simulink subsystem "PvtSubSys_VSM_ELK"  (R2020b)
settings: Solver=VariableStepAuto  StartTime=0.0  StopTime=10.0  RelTol=1e-3
values from neighbouring files (symbols this model uses):
  P_VSM_ELK_Curvature_R_Table : value not decoded    [ELK.sldd]
  P_VSM_ELK_Curvature_R_Table_Calibration : value not decoded    [ELK.sldd]
  P_VSM_ELK_Lane_Width_Table : value not decoded    [ELK.sldd]
  P_VSM_ELK_Lane_Width_Table_Calibration : value not decoded    [ELK.sldd]
  P_VSM_ELK_Lateral_Speed_Table : value not decoded    [ELK.sldd]
  P_VSM_ELK_Lateral_Speed_Table_Calibration : value not decoded    [ELK.sldd]
  P_VSM_ELK_OnComing_Lateral = 2.8    [ELK.sldd]
  P_VSM_ELK_OnComing_TTC = 3.0    [ELK.sldd]
  P_VSM_ELK_OverTaking_Lateral = 2.0    [ELK.sldd]
  P_VSM_ELK_OverTaking_TTC = 5.0    [ELK.sldd]
  P_VSM_ELK_Sensitive_Table : value not decoded    [ELK.sldd]
  P_VSM_ELK_Sensitive_Table_Calibration : value not decoded    [ELK.sldd]
  P_VSM_ELK_State_Absesp_enable = 1.0    [ELK.sldd]
  P_VSM_ELK_State_Accpedalrate_enable = 1.0    [ELK.sldd]
  P_VSM_ELK_State_Breakpressure_enable = 1.0    [ELK.sldd]
  P_VSM_ELK_State_DriverInputTrqValue_enable = 1.0    [ELK.sldd]
  P_VSM_ELK_State_Eps_enable = 1.0    [ELK.sldd]
  P_VSM_ELK_State_ESSSts_enable = 1.0    [ELK.sldd]
  P_VSM_ELK_State_Failsafe_enable = 1.0    [ELK.sldd]
  P_VSM_ELK_State_GEAR_enable = 1.0    [ELK.sldd]
  P_VSM_ELK_State_Handson_enable = 1.0    [ELK.sldd]
  P_VSM_ELK_State_Headingangle_enable = 1.0    [ELK.sldd]
  P_VSM_ELK_State_Lane_enable = 1.0    [ELK.sldd]
  P_VSM_ELK_State_LaneChange_enable = 1.0    [ELK.sldd]
  P_VSM_ELK_State_Lanecurve_enable = 1.0    [ELK.sldd]
  P_VSM_ELK_State_LateralAcce_enable = 1.0    [ELK.sldd]
  P_VSM_ELK_State_LongitudeAcc_enable = 1.0    [ELK.sldd]
  P_VSM_ELK_State_Overide_enable = 1.0    [ELK.sldd]
  P_VSM_ELK_State_Param_AngleOffset = 0.05    [ELK.sldd]
  P_VSM_ELK_State_Param_LaneTime : value not decoded    [ELK.sldd]
  P_VSM_ELK_State_Param_Oncoming = 0.55    [ELK.sldd]
  P_VSM_ELK_State_Param_OnTime : value not decoded    [ELK.sldd]
  P_VSM_ELK_State_Param_OutOffset = 0.15    [ELK.sldd]
  P_VSM_ELK_State_Param_Over = 0.55    [ELK.sldd]
  P_VSM_ELK_State_Param_OvTime : value not decoded    [ELK.sldd]
  P_VSM_ELK_State_Param_Speed : value not decoded    [ELK.sldd]
  P_VSM_ELK_State_SteerWheelAngle_enable = 1.0    [ELK.sldd]
  P_VSM_ELK_State_SteerWheelSpd_enable = 1.0    [ELK.sldd]
  P_VSM_ELK_State_TurnLight_enable = 1.0    [ELK.sldd]
  P_VSM_ELK_State_Vehspeed_enable = 1.0    [ELK.sldd]
  P_VSM_ELK_State_Yawsup_enable = 1.0    [ELK.sldd]
undefined symbols (not defined in the file or in its folder): ELKSTATE, P_Global_DxvRearBumper_m, P_Global_IEnvironment_RefPX_Front_Bumper, P_Global_IFV2Fwheel_Dx, P_Global_Vehicle_Length_m, P_Global_VehicleWidthMin_m, P_VSM_LSMC_SampleTime
libraries: simulink x167
(part 3 of 5)

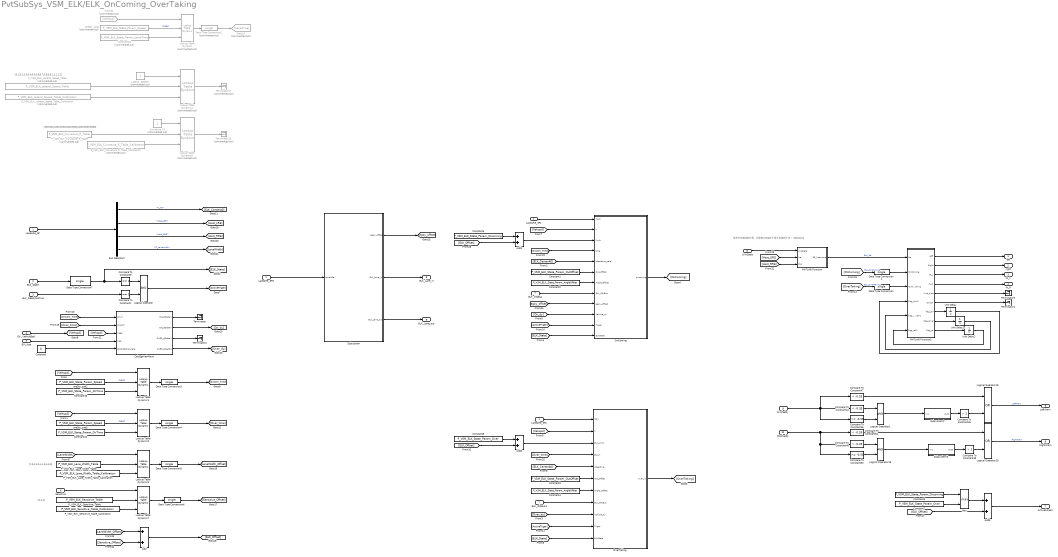
== system PvtSubSys_VSM_ELK/ELK_OnComing_OverTaking ==
  note: 目前对车道线起作用，但是ELKState不显示车道线干涉；
      | 20201011
  note: [0,1,2]
  note: [0.1,0.2,0.3,0.4,0.5,0.6,0.7,0.8,0.9,1,1.1,1.2]
  note: [2.5,3,3.5,4,4.5,5,5.5]
  note: [150,500,1000,1500,2000,3000,4000,5000,5500]
  LaneARe_SP : Inport
  ELK_State : Inport  Port=2
  ELK_Ready2Active : Inport  Port=3
  EVI_VehicleSpd : Inport  Port=4
  EVI_Kap : Inport  Port=5
  Sensitive : Inport  Port=6
  ELK_ObjBus : Inport  Port=7
  LKAState : Inport  Port=8
  FLWhelDy : Inport  Port=9
  FRWhelDy : Inport  Port=10
  Add{,1..3} (4 alike) : Sum
  Bus Selector2 : BusSelector  OutputSignals=T_A0,Host_LRE,Host_RRE,C_Lanewidth
  CalcEgoVehMove : MATLAB Function  TreatAsAtomicUnit=on
  Compare To Constant1 : simulink/Logic and Bit Operations/Compare To Constant  relop===  const=1  OutDataTypeStr=boolean
  Compare To Constant44 : simulink/Logic and Bit Operations/Compare To Constant  relop=<  const=-0.35  OutDataTypeStr=boolean
  Compare To Constant45 : simulink/Logic and Bit Operations/Compare To Constant  relop=>  const=2  OutDataTypeStr=boolean
  Compare To Constant46 : simulink/Logic and Bit Operations/Compare To Constant  relop=>=  const=-0.55  OutDataTypeStr=boolean
  Compare To Constant47 : simulink/Logic and Bit Operations/Compare To Constant  relop=<  const=-0.55  OutDataTypeStr=boolean
  Compare To Constant48 : simulink/Logic and Bit Operations/Compare To Constant  relop=<  const=-0.35  OutDataTypeStr=boolean
  Compare To Constant49 : simulink/Logic and Bit Operations/Compare To Constant  relop=>  const=2  OutDataTypeStr=boolean
  Compare To Constant50 : simulink/Logic and Bit Operations/Compare To Constant  relop=>=  const=-0.55  OutDataTypeStr=boolean
  Compare To Constant51 : simulink/Logic and Bit Operations/Compare To Constant  relop=<  const=-0.55  OutDataTypeStr=boolean
  Compare To Constant9 : simulink/Logic and Bit Operations/Compare To Constant  relop===  const=2  OutDataTypeStr=boolean
  Constant : Constant  Value=0  OutDataTypeStr=single
  Constant1 : Constant  Value=P_VSM_ELK_State_Param_OutOffset
  Constant10 : Constant  Value=P_VSM_ELK_State_Param_OvTime
  Constant15 : Constant  Commented=on  Value=P_VSM_ELK_State_Param_LaneTime
  Constant16 : Constant  Value=P_VSM_ELK_State_Param_OnTime
  Constant2 : Constant  Value=P_VSM_ELK_State_Param_AngleOffset
  Constant3 : Constant  Value=P_VSM_ELK_State_Param_OutOffset
  Constant4 : Constant  Value=P_VSM_ELK_State_Param_AngleOffset
  Constant5 : Constant  Value=P_VSM_ELK_State_Param_Oncoming
  Constant6 : Constant  Value=P_VSM_ELK_State_Param_Oncoming
  Constant7 : Constant  Value=P_VSM_ELK_State_Param_Over
  Constant8 : Constant  Value=P_VSM_ELK_State_Param_Over
  Curvature_R1 : Constant  Commented=on
  Data Type Conversion{,1,3..7} (7 alike) : DataTypeConversion  OutDataTypeStr=single
  Data Type Conversion2 : DataTypeConversion  Commented=on  OutDataTypeStr=single
  ELK_ObjBus1 : InportShadow  Port=7
  From21 : From  Commented=on  GotoTag=VehSpd
  Goto14 : Goto  Commented=on  GotoTag=LaneTime
  LaneARe_SP1 : InportShadow
  LaneARe_SP2 : InportShadow
  LaneARe_SP3 : InportShadow
  Lateral_Speed1 : Constant  Commented=on
  Logical Operator : Logic  AllPortsSameDT=off  OutDataTypeStr=boolean
  Logical Operator1 : Logic  AllPortsSameDT=off  OutDataTypeStr=boolean
  Logical Operator18 : Logic  Operator=OR  AllPortsSameDT=off  OutDataTypeStr=boolean
  Logical Operator19 : Logic  AllPortsSameDT=off  OutDataTypeStr=boolean
  Logical Operator20 : Logic  Operator=OR  AllPortsSameDT=off  OutDataTypeStr=boolean
  Lookup Table Dynamic : simulink/Lookup Tables/Lookup Table Dynamic  Commented=on  LookUpMeth=Interpolation-Use End Values  OutDataType=fixdt('double')  OutScaling=[]  OutputDataTypeScalingMode=Specify via dialog  OutDataTypeStr=double  DoSatur=off
  Lookup Table Dynamic{1..2,5,7} (4 alike) : simulink/Lookup Tables/Lookup Table Dynamic  LookUpMeth=Interpolation-Use End Values  OutDataType=fixdt('double')  OutScaling=[]  OutputDataTypeScalingMode=Specify via dialog  OutDataTypeStr=double  DoSatur=off
  Lookup Table Dynamic4 : simulink/Lookup Tables/Lookup Table Dynamic  Commented=on  LookUpMeth=Interpolation-Use End Values  OutDataType=fixdt('double')  OutScaling=[]  OutputDataTypeScalingMode=Specify via dialog  OutDataTypeStr=double  DoSatur=off
  Lookup Table Dynamic6 : simulink/Lookup Tables/Lookup Table Dynamic  Commented=on  LookUpMeth=Interpolation-Use End Values  OutDataType=fixdt('double')  OutScaling=[]  OutputDataTypeScalingMode=Specify via dialog  OutDataTypeStr=double  DoSatur=off
  MATLAB Function : MATLAB Function  TreatAsAtomicUnit=on
  MATLAB Function2 : MATLAB Function  TreatAsAtomicUnit=on
  Max : MinMax  Function=max  Inputs=2
  OnComing : Subsystem
  OverTaking : Subsystem
  P_VSM_ELK_Curvature_R_Table : Constant  Commented=on  Value=P_VSM_ELK_Curvature_R_Table
  P_VSM_ELK_Curvature_R_Table_Calibration : Constant  Commented=on  Value=P_VSM_ELK_Curvature_R_Table_Calibration
  P_VSM_ELK_Lane_Width_Table : Constant  Value=P_VSM_ELK_Lane_Width_Table
  P_VSM_ELK_Lane_Width_Table_Calibration : Constant  Value=P_VSM_ELK_Lane_Width_Table_Calibration
  P_VSM_ELK_Lateral_Speed_Table : Constant  Commented=on  Value=P_VSM_ELK_Lateral_Speed_Table
  P_VSM_ELK_Lateral_Speed_Table_Calibration : Constant  Commented=on  Value=P_VSM_ELK_Lateral_Speed_Table_Calibration
  P_VSM_ELK_Sensitive_Table : Constant  Value=P_VSM_ELK_Sensitive_Table
  P_VSM_ELK_Sensitive_Table_Calibration : Constant  Value=P_VSM_ELK_Sensitive_Table_Calibration
  Subsystem : Subsystem
  Subsystem2 : Subsystem  mask{Ts=P_VSM_LSMC_SampleTime, Max=10}
      mask prompts: Ts "Sample Time:"; Max "Max Limit:"
      mask Display:
      | Ts=get_param(gcb,'Ts');
      | Max=get_param(gcb,'Max');
      | disp(['Ts:' Ts '\n' 'Max:' Max ]);
  Subsystem3 : Subsystem  mask{Ts=P_VSM_LSMC_SampleTime, Max=10}
      mask prompts: Ts "Sample Time:"; Max "Max Limit:"
      mask Display:
      | Ts=get_param(gcb,'Ts');
      | Max=get_param(gcb,'Max');
      | disp(['Ts:' Ts '\n' 'Max:' Max ]);
  Terminator{,1..3} (4 alike) : Terminator
  Terminator11 : Terminator  Commented=on
  Terminator13 : Terminator  Commented=on
  Unit Delay : UnitDelay  SampleTime=-1  HasFrameUpgradeWarning=on
  Unit Delay1 : UnitDelay  InitialCondition=single(0)  SampleTime=-1  HasFrameUpgradeWarning=on
  Unit Delay2 : UnitDelay  InitialCondition=single(0)  SampleTime=-1  HasFrameUpgradeWarning=on
  preDis_spd1 : Constant  Commented=on  Value=P_VSM_ELK_State_Param_Speed
  preDis_spd2 : Constant  Value=P_VSM_ELK_State_Param_Speed
  preDis_spd3 : Constant  Value=P_VSM_ELK_State_Param_Speed
  "left " : Outport
  "right " : Outport  Port=2
  IN_L : Outport  Port=3
  IN_R : Outport  Port=4
  LeftWarn : Outport  Port=5
  RightWarn : Outport  Port=6
  ActiveZoneIn : Outport  Port=7
  ELK_Lane_in : Outport  Port=8
  ELK_Lane_out : Outport  Port=9
  wires:
  Data Type Conversion7/1 -> [ELK_State], Compare To Constant9/1
  LaneARe_SP2/1 -> OverTaking/1(ican)
  LaneARe_SP1/1 -> OnComing/1(ICAN)
  [On_dy] -> OnComing/10(Vehicle_dy)
  [Over_dy] -> OverTaking/9(Vehicle_dy)
  OverTaking/1("over_in ") -> [OverTaking]
  OnComing/1(oncoming) -> [OnComing]
  ELK_ObjBus1/1 -> OverTaking/8(ELK_ObjBus)
  ELK_ObjBus/1 -> OnComing/8(ELK_ObjBus)
  LKAState/1 -> MATLAB Function/1(LKAState)
  [OnComing] -> Data Type Conversion1/1  "ELK_OnComing"
  [OverTaking] -> Data Type Conversion/1  "ELK_OverTaking"
  MATLAB Function2/6(Switch) -> Terminator1/1
  MATLAB Function2/5(Line_type) -> Terminator3/1
  [egoy_offset] -> OnComing/9(egoy_offset)
  MATLAB Function2/1(Left) -> "left "/1
  MATLAB Function2/2(Right) -> "right "/1
  MATLAB Function2/3(IN_L) -> IN_L/1
  MATLAB Function2/4(IN_R) -> IN_R/1
  Constant1/1 -> OnComing/6(Out_Offset)
  Constant2/1 -> OnComing/7(Angle_Offset)
  [ELK_CenterA0] -> OverTaking/5(Ldeactive)
  Constant3/1 -> OverTaking/6(Out_Offset)
  Constant4/1 -> OverTaking/7(Angle_Offset)
  MATLAB Function2/7(flag_On) -> Unit Delay/1
  MATLAB Function2/8(flag_Over) -> Unit Delay1/1
  MATLAB Function2/9(flag_re) -> Unit Delay2/1
  Unit Delay/1 -> MATLAB Function2/4(flag_Onk1)
  Unit Delay1/1 -> MATLAB Function2/5(flag_Overk1)
  Unit Delay2/1 -> MATLAB Function2/6(flag_rek1)
  MATLAB Function/1(RE_Intervene) -> MATLAB Function2/1(Re)  "ELK_Re"
  [Host_LRE] -> MATLAB Function/2(Lre)
  [Host_RRE] -> MATLAB Function/3(Rre)
  LaneARe_SP/1 -> Bus Selector2/1
  [ELK_CenterA0] -> OnComing/5(Ldeactive_para)
  [ActiveTriger] -> OnComing/11(Triger)
  [ActiveTriger] -> OverTaking/10(Triger)
  Compare To Constant9/1 -> Logical Operator/1
  Compare To Constant1/1 -> Logical Operator/2
  ELK_State/1 -> Data Type Conversion7/1
  ELK_Ready2Active/1 -> Compare To Constant1/1
  Logical Operator/1 -> [ActiveTriger]
  [ELK_State] -> OnComing/12(ELKState)
  [ELK_State] -> OverTaking/11(ELKState)
  Compare To Constant46/1 -> Logical Operator1/2
  Compare To Constant50/1 -> Logical Operator19/2
  Compare To Constant47/1 -> Logical Operator18/1
  Compare To Constant48/1 -> Logical Operator19/1
  Compare To Constant51/1 -> Logical Operator20/1
  FRWhelDy/1 -> Compare To Constant48/1, Compare To Constant50/1, Compare To Constant51/1
  Logical Operator19/1 -> Subsystem3/1(In1)
  Compare To Constant49/1 -> Logical Operator20/2
  Subsystem2/1(Out1) -> Compare To Constant45/1
  Compare To Constant44/1 -> Logical Operator1/1
  Compare To Constant45/1 -> Logical Operator18/2
  FLWhelDy/1 -> Compare To Constant46/1, Compare To Constant47/1, Compare To Constant44/1
  Logical Operator1/1 -> Subsystem2/1(In1)
  Subsystem3/1(Out1) -> Compare To Constant49/1
  Logical Operator18/1 -> LeftWarn/1  "LeftWarn"
  Logical Operator20/1 -> RightWarn/1  "RightWarn"
  Data Type Conversion/1 -> MATLAB Function2/3(OverTaking)
  Data Type Conversion1/1 -> MATLAB Function2/2(OnComing)
  [Vehspd] -> OnComing/2(V)
  [Vehspd] -> OverTaking/2(V)
  EVI_Kap/1 -> CalcEgoVehMove/4(Kap)
  Constant/1 -> CalcEgoVehMove/5(alpSideSlipAngle)
  [Vehspd] -> CalcEgoVehMove/3(Vego)
  [Oncom_Time] -> CalcEgoVehMove/1(On_T)
  [Over_time] -> CalcEgoVehMove/2(Over_T)
  [Oncom_Time] -> OnComing/4(time)
  [Over_time] -> OverTaking/4(ELK_T)
  CalcEgoVehMove/2(ON_dDeltaY) -> [On_dy]
  CalcEgoVehMove/4(OVER_dDeltaY) -> [Over_dy]
  CalcEgoVehMove/1(ON_dDeltaX) -> Terminator/1
  CalcEgoVehMove/3(OVER_dDeltaX) -> Terminator2/1
  EVI_VehicleSpd/1 -> [Vehspd]
  preDis_spd3/1 -> Lookup Table Dynamic2/2  "speed"
  Data Type Conversion3/1 -> [Oncom_Time]
  [Vehspd] -> Lookup Table Dynamic2/1
  preDis_spd1/1 -> Lookup Table Dynamic/2  "speed"
  Lookup Table Dynamic/1 -> Data Type Conversion2/1
  Constant15/1 -> Lookup Table Dynamic/3
  Lookup Table Dynamic1/1 -> Data Type Conversion3/1
  From21/1 -> Lookup Table Dynamic/1
  Constant16/1 -> Lookup Table Dynamic1/3
  Lookup Table Dynamic2/1 -> Data Type Conversion4/1
  Data Type Conversion4/1 -> [Over_time]
  Constant10/1 -> Lookup Table Dynamic2/3
  preDis_spd2/1 -> Lookup Table Dynamic1/2  "speed"
  Data Type Conversion2/1 -> Goto14/1
  [Vehspd] -> Lookup Table Dynamic1/1
  Bus Selector2/1 -> [ELK_CenterA0]  "<T_A0>"
  Constant6/1 -> Add1/1
  [ELK_Offset] -> Add2/2
  [ELK_Offset] -> Add1/2
  Add/1 -> [ELK_Offset]
  Sensitive/1 -> Lookup Table Dynamic7/1
  Data Type Conversion5/1 -> [LaneWidth_Offset]
  P_VSM_ELK_Sensitive_Table/1 -> Lookup Table Dynamic7/2
  Data Type Conversion6/1 -> [Sensitive_Offset]
  [LaneWidth] -> Lookup Table Dynamic5/1
  Lookup Table Dynamic5/1 -> Data Type Conversion5/1
  Lookup Table Dynamic6/1 -> Terminator13/1
  P_VSM_ELK_Lane_Width_Table/1 -> Lookup Table Dynamic5/2
  P_VSM_ELK_Lateral_Speed_Table_Calibration/1 -> Lookup Table Dynamic4/3
  [LaneWidth_Offset] -> Add/1
  P_VSM_ELK_Sensitive_Table_Calibration/1 -> Lookup Table Dynamic7/3
  [Sensitive_Offset] -> Add/2
  P_VSM_ELK_Curvature_R_Table/1 -> Lookup Table Dynamic6/2
  P_VSM_ELK_Curvature_R_Table_Calibration/1 -> Lookup Table Dynamic6/3
  Lookup Table Dynamic4/1 -> Terminator11/1
  Curvature_R1/1 -> Lookup Table Dynamic6/1
  Lateral_Speed1/1 -> Lookup Table Dynamic4/1
  P_VSM_ELK_Lane_Width_Table_Calibration/1 -> Lookup Table Dynamic5/3
  Lookup Table Dynamic7/1 -> Data Type Conversion6/1
  P_VSM_ELK_Lateral_Speed_Table/1 -> Lookup Table Dynamic4/2
  Add1/1 -> OnComing/3(limit)
  Constant8/1 -> Add2/1
  Add2/1 -> OverTaking/3(ELK_Limit)
  Bus Selector2/2 -> [Host_LRE]  "<Host_LRE>"
  Bus Selector2/3 -> [Host_RRE]  "<Host_RRE>"
  Bus Selector2/4 -> [LaneWidth]  "<C_Lanewidth>"
  Constant5/1 -> Max/1
  Constant7/1 -> Max/2
  Max/1 -> Add3/1
  [ELK_Offset] -> Add3/2
  Add3/1 -> ActiveZoneIn/1
  Subsystem/1(egoy_offset) -> [egoy_offset]
  Subsystem/2(ELK_Lane_in) -> ELK_Lane_in/1
  Subsystem/3(ELK_Lane_out) -> ELK_Lane_out/1
  LaneARe_SP3/1 -> Subsystem/1(LaneARe)

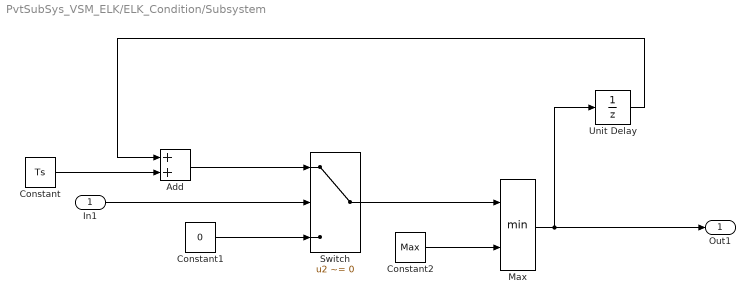
== system PvtSubSys_VSM_ELK/ELK_Condition/Subsystem ==
  In1 : Inport
  Add : Sum
  Constant : Constant  Value=Ts
  Constant1 : Constant  Value=0
  Constant2 : Constant  Value=Max
  Max : MinMax  Inputs=2
  Switch : Switch  Criteria=u2 ~= 0
  Unit Delay : UnitDelay  SampleTime=-1  HasFrameUpgradeWarning=on
  Out1 : Outport
  wires:
  Switch/1 -> Max/1
  Constant2/1 -> Max/2
  Max/1 -> Out1/1, Unit Delay/1
  Add/1 -> Switch/1
  Constant1/1 -> Switch/3
  Constant/1 -> Add/2
  In1/1 -> Switch/2
  Unit Delay/1 -> Add/1

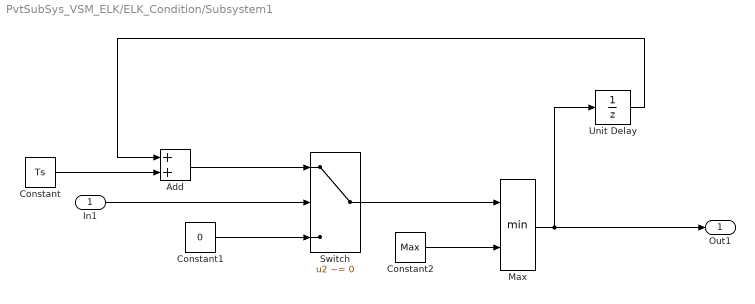
== system PvtSubSys_VSM_ELK/ELK_Condition/Subsystem1 ==
  In1 : Inport
  Add : Sum
  Constant : Constant  Value=Ts
  Constant1 : Constant  Value=0  OutDataTypeStr=single
  Constant2 : Constant  Value=Max  OutDataTypeStr=single
  Max : MinMax  Inputs=2
  Switch : Switch  Criteria=u2 ~= 0
  Unit Delay : UnitDelay  SampleTime=-1  HasFrameUpgradeWarning=on
  Out1 : Outport
  wires:
  Unit Delay/1 -> Add/1
  In1/1 -> Switch/2
  Constant/1 -> Add/2
  Constant1/1 -> Switch/3
  Add/1 -> Switch/1
  Max/1 -> Unit Delay/1, Out1/1
  Constant2/1 -> Max/2
  Switch/1 -> Max/1

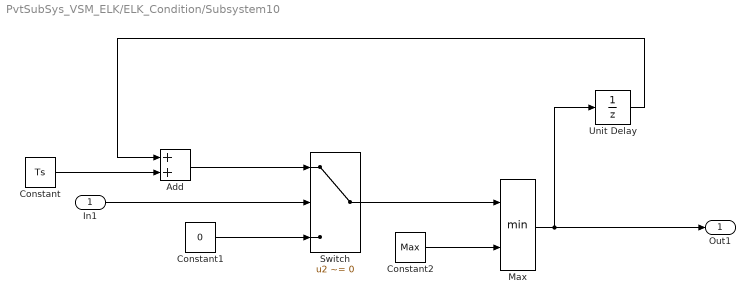
== system PvtSubSys_VSM_ELK/ELK_Condition/Subsystem10 ==
  In1 : Inport
  Add : Sum
  Constant : Constant  Value=Ts
  Constant1 : Constant  Value=0
  Constant2 : Constant  Value=Max
  Max : MinMax  Inputs=2
  Switch : Switch  Criteria=u2 ~= 0
  Unit Delay : UnitDelay  SampleTime=-1  HasFrameUpgradeWarning=on
  Out1 : Outport
  wires:
  Unit Delay/1 -> Add/1
  In1/1 -> Switch/2
  Constant/1 -> Add/2
  Constant1/1 -> Switch/3
  Add/1 -> Switch/1
  Max/1 -> Unit Delay/1, Out1/1
  Constant2/1 -> Max/2
  Switch/1 -> Max/1

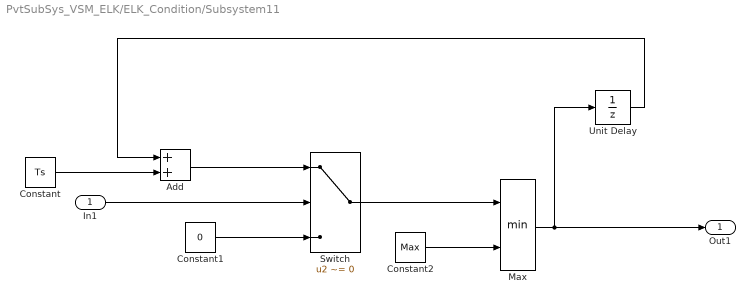
== system PvtSubSys_VSM_ELK/ELK_Condition/Subsystem11 ==
  In1 : Inport
  Add : Sum
  Constant : Constant  Value=Ts
  Constant1 : Constant  Value=0
  Constant2 : Constant  Value=Max
  Max : MinMax  Inputs=2
  Switch : Switch  Criteria=u2 ~= 0
  Unit Delay : UnitDelay  SampleTime=-1  HasFrameUpgradeWarning=on
  Out1 : Outport
  wires:
  Switch/1 -> Max/1
  Constant2/1 -> Max/2
  Max/1 -> Out1/1, Unit Delay/1
  Add/1 -> Switch/1
  Constant1/1 -> Switch/3
  Constant/1 -> Add/2
  In1/1 -> Switch/2
  Unit Delay/1 -> Add/1

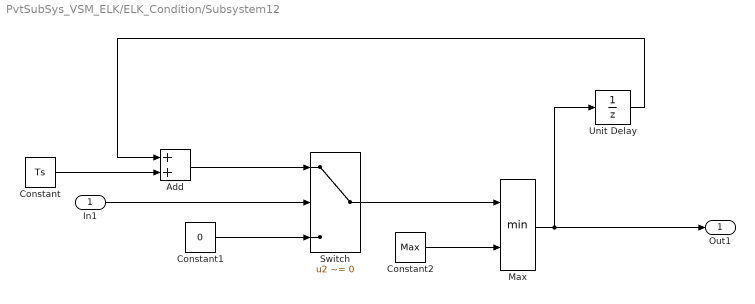
== system PvtSubSys_VSM_ELK/ELK_Condition/Subsystem12 ==
  In1 : Inport
  Add : Sum
  Constant : Constant  Value=Ts
  Constant1 : Constant  Value=0
  Constant2 : Constant  Value=Max
  Max : MinMax  Inputs=2
  Switch : Switch  Criteria=u2 ~= 0
  Unit Delay : UnitDelay  SampleTime=-1  HasFrameUpgradeWarning=on
  Out1 : Outport
  wires:
  Switch/1 -> Max/1
  Constant2/1 -> Max/2
  Max/1 -> Out1/1, Unit Delay/1
  Add/1 -> Switch/1
  Constant1/1 -> Switch/3
  Constant/1 -> Add/2
  In1/1 -> Switch/2
  Unit Delay/1 -> Add/1

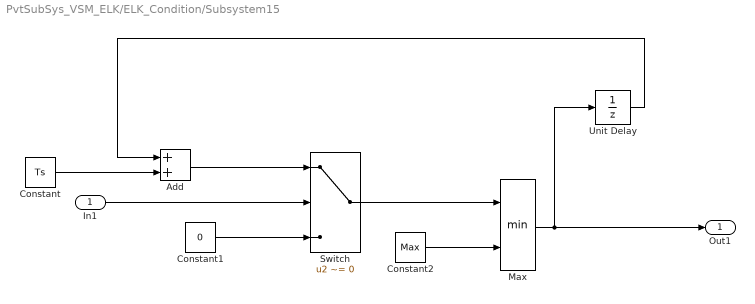
== system PvtSubSys_VSM_ELK/ELK_Condition/Subsystem15 ==
  In1 : Inport
  Add : Sum
  Constant : Constant  Value=Ts
  Constant1 : Constant  Value=0
  Constant2 : Constant  Value=Max
  Max : MinMax  Inputs=2
  Switch : Switch  Criteria=u2 ~= 0
  Unit Delay : UnitDelay  SampleTime=-1  HasFrameUpgradeWarning=on
  Out1 : Outport
  wires:
  Switch/1 -> Max/1
  Constant2/1 -> Max/2
  Max/1 -> Out1/1, Unit Delay/1
  Add/1 -> Switch/1
  Constant1/1 -> Switch/3
  Constant/1 -> Add/2
  In1/1 -> Switch/2
  Unit Delay/1 -> Add/1

== system PvtSubSys_VSM_ELK/ELK_Condition/Subsystem17 ==
  In1 : Inport
  Add : Sum
  Constant : Constant  Value=Ts
  Constant1 : Constant  Value=0
  Constant2 : Constant  Value=Max
  Max : MinMax  Inputs=2
  Switch : Switch  Criteria=u2 ~= 0
  Unit Delay : UnitDelay  SampleTime=-1  HasFrameUpgradeWarning=on
  Out1 : Outport
  wires:
  Unit Delay/1 -> Add/1
  In1/1 -> Switch/2
  Constant/1 -> Add/2
  Constant1/1 -> Switch/3
  Add/1 -> Switch/1
  Max/1 -> Unit Delay/1, Out1/1
  Constant2/1 -> Max/2
  Switch/1 -> Max/1

== system PvtSubSys_VSM_ELK/ELK_Condition/Subsystem2 ==
  In1 : Inport
  Add : Sum
  Constant : Constant  Value=Ts
  Constant1 : Constant  Value=0
  Constant2 : Constant  Value=Max
  Max : MinMax  Inputs=2
  Switch : Switch  Criteria=u2 ~= 0
  Unit Delay : UnitDelay  SampleTime=-1  HasFrameUpgradeWarning=on
  Out1 : Outport
  wires:
  Switch/1 -> Max/1
  Constant2/1 -> Max/2
  Max/1 -> Out1/1, Unit Delay/1
  Add/1 -> Switch/1
  Constant1/1 -> Switch/3
  Constant/1 -> Add/2
  In1/1 -> Switch/2
  Unit Delay/1 -> Add/1

== system PvtSubSys_VSM_ELK/ELK_Condition/Subsystem4 ==
  In1 : Inport
  Add : Sum
  Constant : Constant  Value=Ts
  Constant1 : Constant  Value=0
  Constant2 : Constant  Value=Max
  Max : MinMax  Inputs=2
  Switch : Switch  Criteria=u2 ~= 0
  Unit Delay : UnitDelay  SampleTime=-1  HasFrameUpgradeWarning=on
  Out1 : Outport
  wires:
  Unit Delay/1 -> Add/1
  In1/1 -> Switch/2
  Constant/1 -> Add/2
  Constant1/1 -> Switch/3
  Add/1 -> Switch/1
  Max/1 -> Unit Delay/1, Out1/1
  Constant2/1 -> Max/2
  Switch/1 -> Max/1

== system PvtSubSys_VSM_ELK/ELK_Condition/Subsystem5 ==
  In1 : Inport
  Add : Sum
  Constant : Constant  Value=Ts
  Constant1 : Constant  Value=0
  Constant2 : Constant  Value=Max
  Max : MinMax  Inputs=2
  Switch : Switch  Criteria=u2 ~= 0
  Unit Delay : UnitDelay  SampleTime=-1  HasFrameUpgradeWarning=on
  Out1 : Outport
  wires:
  Switch/1 -> Max/1
  Constant2/1 -> Max/2
  Max/1 -> Out1/1, Unit Delay/1
  Add/1 -> Switch/1
  Constant1/1 -> Switch/3
  Constant/1 -> Add/2
  In1/1 -> Switch/2
  Unit Delay/1 -> Add/1

== system PvtSubSys_VSM_ELK/ELK_Condition/Subsystem6 ==
  In1 : Inport
  Add : Sum
  Constant : Constant  Value=Ts
  Constant1 : Constant  Value=0
  Constant2 : Constant  Value=Max
  Max : MinMax  Inputs=2
  Switch : Switch  Criteria=u2 ~= 0
  Unit Delay : UnitDelay  SampleTime=-1  HasFrameUpgradeWarning=on
  Out1 : Outport
  wires:
  Switch/1 -> Max/1
  Constant2/1 -> Max/2
  Max/1 -> Out1/1, Unit Delay/1
  Add/1 -> Switch/1
  Constant1/1 -> Switch/3
  Constant/1 -> Add/2
  In1/1 -> Switch/2
  Unit Delay/1 -> Add/1

== system PvtSubSys_VSM_ELK/ELK_Condition/Subsystem7 ==
  In1 : Inport
  Add : Sum
  Constant : Constant  Value=Ts
  Constant1 : Constant  Value=0
  Constant2 : Constant  Value=Max
  Max : MinMax  Inputs=2
  Switch : Switch  Criteria=u2 ~= 0
  Unit Delay : UnitDelay  SampleTime=-1  HasFrameUpgradeWarning=on
  Out1 : Outport
  wires:
  Unit Delay/1 -> Add/1
  In1/1 -> Switch/2
  Constant/1 -> Add/2
  Constant1/1 -> Switch/3
  Add/1 -> Switch/1
  Max/1 -> Unit Delay/1, Out1/1
  Constant2/1 -> Max/2
  Switch/1 -> Max/1

== system PvtSubSys_VSM_ELK/ELK_Condition/Subsystem8 ==
  In1 : Inport
  Add : Sum
  Constant : Constant  Value=Ts
  Constant1 : Constant  Value=0
  Constant2 : Constant  Value=Max
  Max : MinMax  Inputs=2
  Switch : Switch  Criteria=u2 ~= 0
  Unit Delay : UnitDelay  SampleTime=-1  HasFrameUpgradeWarning=on
  Out1 : Outport
  wires:
  Unit Delay/1 -> Add/1
  In1/1 -> Switch/2
  Constant/1 -> Add/2
  Constant1/1 -> Switch/3
  Add/1 -> Switch/1
  Max/1 -> Unit Delay/1, Out1/1
  Constant2/1 -> Max/2
  Switch/1 -> Max/1

== system PvtSubSys_VSM_ELK/ELK_Condition/Subsystem9 ==
  In1 : Inport
  Add : Sum
  Constant : Constant  Value=Ts
  Constant1 : Constant  Value=0
  Constant2 : Constant  Value=Max
  Max : MinMax  Inputs=2
  Switch : Switch  Criteria=u2 ~= 0
  Unit Delay : UnitDelay  SampleTime=-1  HasFrameUpgradeWarning=on
  Out1 : Outport
  wires:
  Switch/1 -> Max/1
  Constant2/1 -> Max/2
  Max/1 -> Out1/1, Unit Delay/1
  Add/1 -> Switch/1
  Constant1/1 -> Switch/3
  Constant/1 -> Add/2
  In1/1 -> Switch/2
  Unit Delay/1 -> Add/1

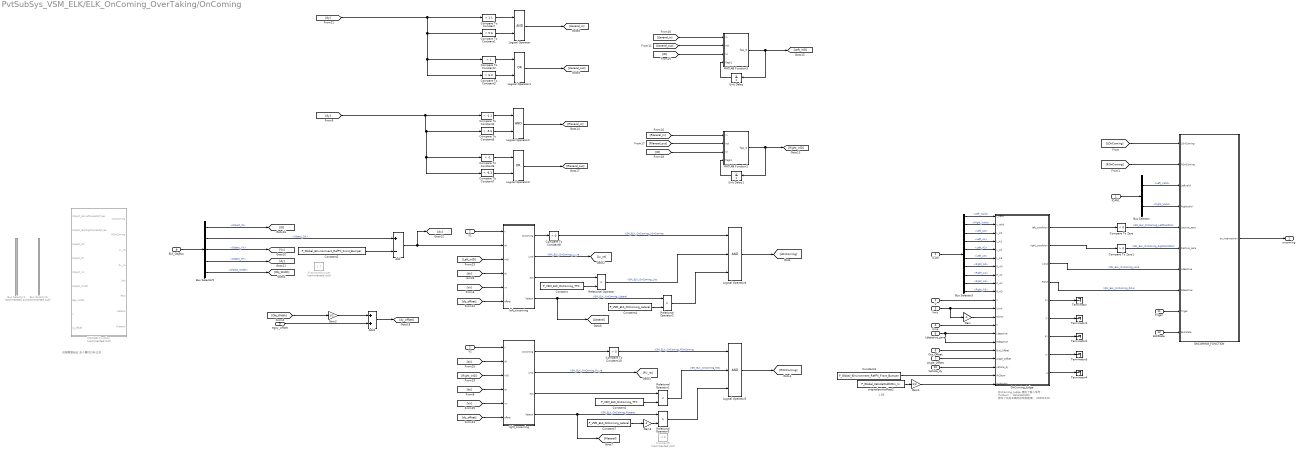
== system PvtSubSys_VSM_ELK/ELK_OnComing_OverTaking/OnComing ==
  note: OnComing_Judge
      | 增加了输入信号：
      | ifv2bum；
      | VehicleWidth;
      | 修改了自车车辆动态预测距离；
      | 20201010
  note: 后期需要验证 各个属性方向/正负
  note: 1.86
  ICAN : Inport
  V : Inport  Port=2
  limit : Inport  Port=3
  time : Inport  Port=4
  Ldeactive_para : Inport  Port=5
  Out_Offset : Inport  Port=6
  Angle_Offset : Inport  Port=7
  ELK_ObjBus : Inport  Port=8
  egoy_offset : Inport  Port=9
  Vehicle_dy : Inport  Port=10
  Triger : Inport  Port=11
  ELKState : Inport  Port=12
  Add : Sum  Inputs=+-
  Add1 : Sum
  Bus Selector : BusSelector  OutputSignals=Left_Valid,Right_Valid
  Bus Selector1 : BusSelector  Commented=on  OutputSignals=ELK_Object_ID,ELK_Object_DX,ELK_Object_VX,ELK_Object_DY,ELK_Object_Width
  Bus Selector3 : BusSelector  OutputSignals=Left_Valid,Right_Valid,Left_A0,Left_A1,Left_A2,Left_A3,Right_A0,Right_A1,Right_A2,Right_A3
  Bus Selector5 : BusSelector  OutputSignals=Object_ID,Object_DX,Object_VX,Object_DY,Object_Width
  Bus Selector6 : BusSelector  Commented=on  OutputSignals=IFC_ID,Long_Pos,Long_Vel,Lat_Pos,VIS_OBS_WIDTH
  Compare To Constant : simulink/Logic and Bit Operations/Compare To Constant  relop=>  const=1.1  OutDataTypeStr=boolean
  Compare To Constant1 : simulink/Logic and Bit Operations/Compare To Constant  relop=<  const=5.6  OutDataTypeStr=boolean
  Compare To Constant10 : simulink/Logic and Bit Operations/Compare To Constant  relop=>  const=0  OutDataTypeStr=boolean
  Compare To Constant2 : simulink/Logic and Bit Operations/Compare To Constant  relop=<  const=1  OutDataTypeStr=boolean
  Compare To Constant3 : simulink/Logic and Bit Operations/Compare To Constant  relop=>  const=6.3  OutDataTypeStr=boolean
  Compare To Constant4 : simulink/Logic and Bit Operations/Compare To Constant  relop=<  const=-1.1  OutDataTypeStr=boolean
  Compare To Constant5 : simulink/Logic and Bit Operations/Compare To Constant  relop=>  const=-5.6  OutDataTypeStr=boolean
  Compare To Constant6 : simulink/Logic and Bit Operations/Compare To Constant  relop=>  const=-1  OutDataTypeStr=boolean
  Compare To Constant7 : simulink/Logic and Bit Operations/Compare To Constant  relop=<  const=-6.3  OutDataTypeStr=boolean
  Compare To Constant8 : simulink/Logic and Bit Operations/Compare To Constant  relop=>  const=0  OutDataTypeStr=boolean
  Compare To Zero : simulink/Logic and Bit Operations/Compare To Zero  relop=<  OutDataTypeStr=boolean
  Compare To Zero1 : simulink/Logic and Bit Operations/Compare To Zero  relop=>  OutDataTypeStr=boolean
  Constant : Constant  Value=P_VSM_ELK_OnComing_TTC
  Constant1 : Constant  Value=P_VSM_ELK_OnComing_TTC
  Constant2 : Constant  Value=P_Global_IEnvironment_RefPX_Front_Bumper
  Constant3 : Constant  Value=P_Global_IEnvironment_RefPX_Front_Bumper
  Constant4 : Constant  Value=P_VSM_ELK_OnComing_Lateral
  Constant5 : Constant  Commented=on  Value=-2.8
  Constant7 : Constant  Value=P_VSM_ELK_OnComing_Lateral
  Gain : Gain  Gain=-1
  Gain1 : Gain  Gain=1/2
  Gain2 : Gain  Gain=1/2
  Gain3 : Gain  Gain=-1
  ICAN1 : InportShadow
  Logical Operator : Logic  AllPortsSameDT=off  OutDataTypeStr=boolean
  Logical Operator1 : Logic  Operator=OR  AllPortsSameDT=off  OutDataTypeStr=boolean
  Logical Operator2 : Logic  AllPortsSameDT=off  OutDataTypeStr=boolean
  Logical Operator3 : Logic  Operator=OR  AllPortsSameDT=off  OutDataTypeStr=boolean
  Logical Operator4 : Logic  Inputs=3  AllPortsSameDT=off  OutDataTypeStr=boolean
  Logical Operator5 : Logic  Inputs=3  AllPortsSameDT=off  OutDataTypeStr=boolean
  MATLAB Function : MATLAB Function  Commented=on  TreatAsAtomicUnit=on
  MATLAB Function1 : MATLAB Function  TreatAsAtomicUnit=on
  MATLAB Function3 : MATLAB Function  TreatAsAtomicUnit=on
  ONCOMING_FUNCTION : Stateflow chart  TreatAsAtomicUnit=on
  OnComing_Judge : MATLAB Function  TreatAsAtomicUnit=on
  Relational Operator : RelationalOperator  Operator=<  OutDataTypeStr=boolean  RndMeth=Simplest
  Relational Operator1 : RelationalOperator  Operator=<  OutDataTypeStr=boolean  RndMeth=Simplest
  Relational Operator2 : RelationalOperator  Operator=<  OutDataTypeStr=boolean  RndMeth=Simplest
  Relational Operator3 : RelationalOperator  Operator=>  OutDataTypeStr=boolean  RndMeth=Simplest
  Terminator{,1..4} (5 alike) : Terminator
  Unit Delay : UnitDelay  InitialCondition=uint8(0)  SampleTime=-1  HasFrameUpgradeWarning=on
  Unit Delay1 : UnitDelay  InitialCondition=uint8(0)  SampleTime=-1  HasFrameUpgradeWarning=on
  V1 : InportShadow  Port=2
  V2 : InportShadow  Port=2
  ifvtofrontbumper : Constant  Commented=on  Value=1.7
  left_oncoming : MATLAB Function  TreatAsAtomicUnit=on
  originalpointoffset2 : Constant  Value=P_Global_VehicleWidthMin_m
  right_oncoming : MATLAB Function  TreatAsAtomicUnit=on
  oncoming : Outport
  wires:
  Bus Selector/2 -> ONCOMING_FUNCTION/4(Rightvalid)  "<Right_Valid>"
  Bus Selector/1 -> ONCOMING_FUNCTION/3(Leftvalid)  "<Left_Valid>"
  ICAN1/1 -> Bus Selector/1
  Bus Selector3/10 -> OnComing_Judge/10(R_A3)  "<Right_A3>"
  Bus Selector3/9 -> OnComing_Judge/9(R_A2)  "<Right_A2>"
  Bus Selector3/8 -> OnComing_Judge/8(R_A1)  "<Right_A1>"
  Bus Selector3/7 -> OnComing_Judge/7(R_A0)  "<Right_A0>"
  Bus Selector3/6 -> OnComing_Judge/6(L_A3)  "<Left_A3>"
  Bus Selector3/5 -> OnComing_Judge/5(L_A2)  "<Left_A2>"
  Bus Selector3/4 -> OnComing_Judge/4(L_A1)  "<Left_A1>"
  Bus Selector3/3 -> OnComing_Judge/3(L_A0)  "<Left_A0>"
  Bus Selector3/2 -> OnComing_Judge/2(r_valid)  "<Right_Valid>"
  Bus Selector3/1 -> OnComing_Judge/1(l_valid)  "<Left_Valid>"
  Gain3/1 -> Relational Operator3/2
  OnComing_Judge/9(a) -> Terminator4/1
  [Vx] -> left_oncoming/5(vx)
  Bus Selector5/5 -> [Obj_Width]  "<Object_Width>"
  Bus Selector5/3 -> [Vx]  "<Object_VX>"
  Bus Selector5/2 -> Add/1  "<Object_DX>"
  Bus Selector5/1 -> [ID]  "<Object_ID>"
  ELK_ObjBus/1 -> Bus Selector5/1
  Unit Delay1/1 -> MATLAB Function1/4(flagk1)
  Unit Delay/1 -> MATLAB Function3/4(flagk1)
  Constant1/1 -> Relational Operator1/2
  Constant/1 -> Relational Operator/2
  Angle_Offset/1 -> OnComing_Judge/18(Angle_Offset)
  Out_Offset/1 -> OnComing_Judge/17(Out_Offset)
  OnComing_Judge/4(ROut) -> ONCOMING_FUNCTION/8(Rdeactive)  "VSM_ELK_OnComing_ROut"
  OnComing_Judge/3(LOut) -> ONCOMING_FUNCTION/7(Ldeactive)  "VSM_ELK_OnComing_LOut"
  OnComing_Judge/2(right_condition) -> Compare To Zero1/1
  OnComing_Judge/1(left_condition) -> Compare To Zero/1
  Ldeactive_para/1 -> OnComing_Judge/16(Rdeactive), OnComing_Judge/15(Ldeactive)
  [ROnComing] -> ONCOMING_FUNCTION/2(ROnComing)
  [LOnComing] -> ONCOMING_FUNCTION/1(LOnComing)
  Logical Operator5/1 -> [ROnComing]
  Logical Operator4/1 -> [LOnComing]
  Relational Operator1/1 -> Logical Operator5/2  "VSM_ELK_OnComing_Rttc"
  Compare To Constant10/1 -> Logical Operator5/1  "VSM_ELK_OnComing_ROnComing"
  Relational Operator/1 -> Logical Operator4/2  "VSM_ELK_OnComing_Lttc"
  Compare To Constant8/1 -> Logical Operator4/1  "VSM_ELK_OnComing_LOnComing"
  [dy_offset] -> right_oncoming/6(offset)
  [dy_offset] -> left_oncoming/6(offset)
  Add1/1 -> [dy_offset]
  egoy_offset/1 -> Add1/2
  Gain2/1 -> Add1/1
  [Obj_Width] -> Gain2/1
  [dx] -> right_oncoming/2(dx)
  [Vx] -> right_oncoming/5(vx)
  [Right_inID] -> right_oncoming/3(inID)
  Compare To Constant4/1 -> Logical Operator2/1
  MATLAB Function1/1(flag_id) -> [Right_inID], Unit Delay1/1
  [ID] -> MATLAB Function1/3(id)
  Compare To Constant5/1 -> Logical Operator2/2
  Compare To Constant7/1 -> Logical Operator3/2
  Logical Operator2/1 -> [Rlareral_in]
  Compare To Constant6/1 -> Logical Operator3/1
  [dy] -> Compare To Constant7/1, Compare To Constant6/1, Compare To Constant5/1, Compare To Constant4/1
  Logical Operator3/1 -> [Rlareral_out]
  [Rlareral_in] -> MATLAB Function1/1(in)
  [Rlareral_out] -> MATLAB Function1/2(out)
  [dy] -> right_oncoming/4(dy)
  Bus Selector5/4 -> [dy]  "<Object_DY>"
  [Llareral_out] -> MATLAB Function3/2(out)
  [Llareral_in] -> MATLAB Function3/1(in)
  [Left_inID] -> left_oncoming/3(inID)
  Logical Operator1/1 -> [Llareral_out]
  [dy] -> Compare To Constant/1, Compare To Constant1/1, Compare To Constant2/1, Compare To Constant3/1
  Compare To Constant2/1 -> Logical Operator1/1
  Logical Operator/1 -> [Llareral_in]
  Compare To Constant3/1 -> Logical Operator1/2
  Compare To Constant1/1 -> Logical Operator/2
  [ID] -> MATLAB Function3/3(id)
  MATLAB Function3/1(flag_id) -> [Left_inID], Unit Delay/1
  Add/1 -> left_oncoming/2(dx), [dx]
  Compare To Constant/1 -> Logical Operator/1
  left_oncoming/4(llateral) -> Relational Operator2/1, [Llateral]  "VSM_ELK_OnComing_Llateral"
  V2/1 -> right_oncoming/1(v)
  V1/1 -> left_oncoming/1(v)
  [dy] -> left_oncoming/4(dy)
  right_oncoming/4(llateral) -> Relational Operator3/1, [Rlateral]  "VSM_ELK_OnComing_Rlateral"
  right_oncoming/3(lttc) -> Relational Operator1/1
  right_oncoming/2(lvrel) -> [Rv_re]  "VSM_ELK_OnComing_Rv_re"
  right_oncoming/1(oncoming) -> Compare To Constant10/1
  left_oncoming/3(lttc) -> Relational Operator/1
  left_oncoming/2(lvrel) -> [Lv_re]  "VSM_ELK_OnComing_Lv_re"
  left_oncoming/1(oncoming) -> Compare To Constant8/1
  ONCOMING_FUNCTION/1(on_intervention) -> oncoming/1
  Gain/1 -> OnComing_Judge/13(Rlimit)
  ICAN/1 -> Bus Selector3/1
  limit/1 -> Gain/1, OnComing_Judge/12(Limit)
  V/1 -> OnComing_Judge/11(V)
  time/1 -> OnComing_Judge/14(T)
  Vehicle_dy/1 -> OnComing_Judge/19(vehicle_dy)
  Compare To Zero/1 -> ONCOMING_FUNCTION/5(Lactive_para)  "VSM_ELK_OnComing_LetfCondition"
  Compare To Zero1/1 -> ONCOMING_FUNCTION/6(Ractive_para)  "VSM_ELK_OnComing_RightCondition"
  Constant2/1 -> Add/2
  originalpointoffset2/1 -> Gain1/1
  Gain1/1 -> OnComing_Judge/21(HalfWidth)
  Constant3/1 -> OnComing_Judge/20(ifv2bum)
  OnComing_Judge/5(LY) -> Terminator/1
  OnComing_Judge/6(ly) -> Terminator1/1
  OnComing_Judge/7(RY) -> Terminator2/1
  OnComing_Judge/8(ry) -> Terminator3/1
  Triger/1 -> ONCOMING_FUNCTION/9(Triger)
  Relational Operator2/1 -> Logical Operator4/3
  Constant4/1 -> Relational Operator2/2
  ELKState/1 -> ONCOMING_FUNCTION/10(ELKState)
  Constant7/1 -> Gain3/1
  Relational Operator3/1 -> Logical Operator5/3
